simulink model "Final_Model_Building_2_AirflowAdded_BufferMode"  (R2022a)
settings: Solver=FixedStepAuto  StartTime=0.0  StopTime=24*3600  FixedStep=5  RelTol=1e-3
values from neighbouring files (symbols this model uses):
  Aux_Threshold = 52    [Setup_Code_EWASP_VC.m]
  buildingAge = 2005    [Setup_Code_EWASP_VC.m]
  ceilingHeight = 2.4    [Setup_Code_EWASP_VC.m]
  conductiveHconnectMatrix = [ ... (first row only)    [Setup_Code_EWASP_VC.m]
  cRoofGreen = 100000    [Setup_Code_EWASP_VC.m]
  Defrost_After_Time = 30    [Setup_Code_EWASP_VC.m]
  DHWDemandProfile = occFreegainHotwaterElecTestPassiveOcc3(:,3)    [Setup_Code_EWASP_VC.m]
  Elec_Max = Elec_Max*(30/24.2)    [Setup_Code_EWASP_VC.m]
  Elec_Mid = Elec_Mid*(30/24.2)    [Setup_Code_EWASP_VC.m]
  Elec_Min = Elec_Min*(30/24.2)    [Setup_Code_EWASP_VC.m]
  ElecDemandProfile = occFreegainHotwaterElecTestPassiveOcc3(:,4)    [Setup_Code_EWASP_VC.m]
  ElecFixed = [Elec_Max(6,2) Elec_Max(6,4) Elec_Max(6,6) Elec_Max(6,7) ... (first row only)    [Setup_Code_EWASP_VC.m]
  floorOrCeilingArea = floorOrCeilingArea*1.15    [Setup_Code_EWASP_VC.m]
  freegain = occFreegainHotwaterElecTestPassiveOcc3(:,2)-max(occupancy)*25    [Setup_Code_EWASP_VC.m]
  furnitureModelOn = 1    [Setup_Code_EWASP_VC.m]
  Heat_Max = Heat_Max*(30/24.2)    [Setup_Code_EWASP_VC.m]
  Heat_Mid = Heat_Mid*(30/24.2)    [Setup_Code_EWASP_VC.m]
  Heat_Min = Heat_Min*(30/24.2)    [Setup_Code_EWASP_VC.m]
  HeatFixed = [Heat_Max(6,2) Heat_Max(6,4) Heat_Max(6,6) Heat_Max(6,7) ... (first row only)    [Setup_Code_EWASP_VC.m]
  HeatingOnProfile = repmat(HeatingOnProfile,365,1)    [Setup_Code_EWASP_VC.m]
  HEX_ReturnLowerLimit = 52.5    [Setup_Code_EWASP_VC.m]
  HEX_ReturnUpperLimit = 55    [Setup_Code_EWASP_VC.m]
  LeakMultiplier = 1+(2*(rand()-0.5)/10)    [Setup_Code_EWASP_VC.m]
  maxOcc = max(occupancyProfile)    [Setup_Code_EWASP_VC.m]
  NESW_wallArea = max(NESW_Lengths*ceilingHeight-NESW_Windows,0)    [Setup_Code_EWASP_VC.m]
  NESW_Windows = [ ... (first row only)    [Setup_Code_EWASP_VC.m]
  numRooms = roomCount    [Setup_Code_EWASP_VC.m]
  occupancy = occupancyProfile    [Setup_Code_EWASP_VC.m]
  offsetDays = 0    [Setup_Code_EWASP_VC.m]
  overChargeSeries = repmat(overChargeSeries,365,1)    [Setup_Code_EWASP_VC.m]
  pumpChoice = pumpChoices(MinIndex,1)    [Setup_Code_EWASP_VC.m]
  pumpRamp = 180    [Setup_Code_EWASP_VC.m]
  RoofIrradiance = Flat_NS_EW_RoofIrradiance(:,1)    [Setup_Code_EWASP_VC.m]
  roofStartTemp = ones(11,1)*20    [Setup_Code_EWASP_VC.m]
  rooftype = 0    [Setup_Code_EWASP_VC.m]
  RoomDataMatrix = [zeros(1,12);ones(1,12)*wallDensity;zeros(1,12);ones(1,12)*wallU;ones(1,12)*windowU;ones(1,12)*floorU;ones(1,12)*ceilingU;zeros(1,12);windowArea, 0;floorOrCeilingArea;zeros(1,12);floorOrCeilingArea*ceilingHeight]    [Setup_Code_EWASP_VC.m]
  roomVol = roomVol*1.15    [Setup_Code_EWASP_VC.m]
  slabStartTemp = (GroundTempTimeSeries(offsetDays*1440+1,1)+thermostatSetting)/2    [Setup_Code_EWASP_VC.m]
  SlackRequest = zeros(1440,1)    [Setup_Code_EWASP_VC.m]
  SolarThermalExists = 0    [Setup_Code_EWASP_VC.m]
  SourceFixed = HeatFixed-ElecFixed    [Setup_Code_EWASP_VC.m]
  StateSeries = StateSeriesGenerator(22,7,1)    [Setup_Code_EWASP_VC.m]
  Tank_Lower_Temp = 49.5    [Setup_Code_EWASP_VC.m]
  Tank_Upper_Temp = 52    [Setup_Code_EWASP_VC.m]
  Tank_Volume_m3 = 0.15    [Setup_Code_EWASP_VC.m]
  TankHeatHour = randi([1 5])-1    [Setup_Code_EWASP_VC.m]
  upDown = [0;0;0;0;1;1;1;1;1;1;1]    [Setup_Code_EWASP_VC.m]
  wallStartTempExt = thermostatSetting*(0.266+0.00215*outdoorStartTemp+0.018*wallU+0.00113*outdoorStartTemp*wallU+0.0068*wallU^2)    [Setup_Code_EWASP_VC.m]
undefined symbols (not defined in the file or in its folder): a, ceilingU, condUDMatrix, convUDMatrix, deltaPEXPANDED_E, deltaPEXPANDED_E2, deltaPEXPANDED_N, deltaPEXPANDED_N2, deltaPEXPANDED_S, deltaPEXPANDED_S2, deltaPEXPANDED_W, deltaPEXPANDED_W2, DesiredDHWTemp, DesiredFlowTempVsInOutDeltaTemp, DiffuseHorizontal, DiscIntNeverNeededParam, DNI, dwnAndConcrete, ExtractRates, GroundTempTimeSeries, HCM, HCM2, HCM_closed, HCM_closed2, intermediateU, IsTop, massFlowMatrix, mechEfficiency, neighbourMatrix, numericalRoomUse, RadiatorMatrix, room2roomflowmatrix_E, room2roomflowmatrix_E2, room2roomflowmatrix_N, room2roomflowmatrix_N2, room2roomflowmatrix_S, room2roomflowmatrix_S2, room2roomflowmatrix_W, room2roomflowmatrix_W2, StateAirInEXPANDED_E, StateAirInEXPANDED_E2, StateAirInEXPANDED_N, StateAirInEXPANDED_N2, StateAirInEXPANDED_S, StateAirInEXPANDED_S2, StateAirInEXPANDED_W, StateAirInEXPANDED_W2, StateAirOutEXPANDED_E, StateAirOutEXPANDED_E2, StateAirOutEXPANDED_N, StateAirOutEXPANDED_N2, StateAirOutEXPANDED_S, StateAirOutEXPANDED_S2, StateAirOutEXPANDED_W, StateAirOutEXPANDED_W2, tankExists, TemperatureSeries, ThermostatBand, ThermostatSetting, Tin1 ... (+10)
libraries: simulink x6, dspsigops x4, dspmtrx3 x4, powerlib_meascontrol x3, carnot x3, dspstat3 x2
(part 29 of 29)

== matlab function Final_Model_Building_2_AirflowAdded_BufferMode/Subsystem_Room6/Bedroom1/Subsystem3/MATLAB Function ==
  data: uValWall input; deltaTint output; c_InPU input; c_MidPU input; c_OutPU input; T_InWall input; T_MidWall input; T_OutWall input; T_Room input; T_AmbientSeries input; windSpeedSeries input; deltaTmid output; deltaTout output; ceilArea input; roomNumber input; logRoomHeatLoss output; Time input; offsetDays input
function [deltaTint,deltaTmid,deltaTout,logRoomHeatLoss] = fcn(uValWall,c_InPU,c_MidPU,c_OutPU,T_InWall, T_MidWall,T_OutWall,T_Room,T_AmbientSeries,windSpeedSeries,ceilArea,roomNumber,Time,offsetDays)




  deltaTint=zeros(1,1);
   deltaTmid=zeros(1,1);
    deltaTout=zeros(1,1);
    logRoomHeatLoss=zeros(1,1);

    v_Wind=windSpeedSeries(ceil((offsetDays*1440)+Time/60+0.00001),1);
   T_Ambient=T_AmbientSeries(ceil((offsetDays*1440)+Time/60+0.00001),1);
    
k_InMid=uValWall*2;
k_OutMid=uValWall*2;




    
    if ceilArea>0

c_In=c_InPU*ceilArea;
c_Mid=c_MidPU*ceilArea;
c_Out=c_OutPU*ceilArea;

    
aA=[-(k_InMid*ceilArea)/c_In (k_InMid*ceilArea)/c_In 0
 (k_InMid*ceilArea)/c_Mid -((k_InMid+k_OutMid)*ceilArea)/c_Mid (k_OutMid*ceilArea)/c_Mid
 0 (k_OutMid*ceilArea)/c_Out -(k_OutMid*ceilArea)/c_Out];

bA=[1/c_In 0 0
 0 1/c_Mid 0
 0 0 1/c_Out];
    
ab=[T_InWall
    T_MidWall
    T_OutWall];

bb=[(2.5*(T_Room-T_InWall)+5.6*(T_Room-T_InWall))*ceilArea
0    
(2.8+3*v_Wind)*(T_Ambient-T_OutWall)+5.6*(T_Ambient-T_OutWall)*ceilArea];

deltaT=aA*ab+bA*bb;

    deltaTint=deltaT(1,1);
   deltaTmid=deltaT(2,1);
    deltaTout=deltaT(3,1);
    
    logRoomHeatLoss=bb(1,1);
    
    else
        
        deltaTint=0;
   deltaTmid=0;
    deltaTout=0;
        
    logRoomHeatLoss=0;
    
    end

== matlab function Final_Model_Building_2_AirflowAdded_BufferMode/Subsystem_Room6/Bedroom1/Subsystem3/MATLAB Function1 ==
  data: Time input; offsetDays input; SurfaceAlbedo input; Tot_Irradiance output; RoofArea input; c_OutRoof input; deltaTexternal output; RoofIrradiance input
function [Tot_Irradiance, deltaTexternal] = SolarSeriesToExtWallGains(Time,offsetDays,SurfaceAlbedo,RoofArea,c_OutRoof,RoofIrradiance)

PU_AreaIrr=RoofIrradiance(ceil((offsetDays*1440)+Time/60+0.00001),1)/2;%extracts correct Diff for the timestep, factor of 1/2 corrects for 90 degree walls (so only half Diff irradiance can be utilised)


Tot_Irradiance=(RoofArea*PU_AreaIrr)*(1-SurfaceAlbedo);
deltaTexternal=Tot_Irradiance./(c_OutRoof*RoofArea);

    
end

== matlab function Final_Model_Building_2_AirflowAdded_BufferMode/Subsystem_Room2/Kitchen/Subsystem3/MATLAB Function ==
  data: uValWall input; deltaTint output; c_InPU input; c_MidPU input; c_OutPU input; T_InWall input; T_MidWall input; T_OutWall input; T_Room input; T_AmbientSeries input; windSpeedSeries input; deltaTmid output; deltaTout output; ceilArea input; roomNumber input; logRoomHeatLoss output; Time input; offsetDays input
function [deltaTint,deltaTmid,deltaTout,logRoomHeatLoss] = fcn(uValWall,c_InPU,c_MidPU,c_OutPU,T_InWall, T_MidWall,T_OutWall,T_Room,T_AmbientSeries,windSpeedSeries,ceilArea,roomNumber,Time,offsetDays)




  deltaTint=zeros(1,1);
   deltaTmid=zeros(1,1);
    deltaTout=zeros(1,1);
    logRoomHeatLoss=zeros(1,1);

    v_Wind=windSpeedSeries(ceil((offsetDays*1440)+Time/60+0.00001),1);
   T_Ambient=T_AmbientSeries(ceil((offsetDays*1440)+Time/60+0.00001),1);
    
k_InMid=uValWall*2;
k_OutMid=uValWall*2;




    
    if ceilArea>0

c_In=c_InPU*ceilArea;
c_Mid=c_MidPU*ceilArea;
c_Out=c_OutPU*ceilArea;

    
aA=[-(k_InMid*ceilArea)/c_In (k_InMid*ceilArea)/c_In 0
 (k_InMid*ceilArea)/c_Mid -((k_InMid+k_OutMid)*ceilArea)/c_Mid (k_OutMid*ceilArea)/c_Mid
 0 (k_OutMid*ceilArea)/c_Out -(k_OutMid*ceilArea)/c_Out];

bA=[1/c_In 0 0
 0 1/c_Mid 0
 0 0 1/c_Out];
    
ab=[T_InWall
    T_MidWall
    T_OutWall];

bb=[(2.5*(T_Room-T_InWall)+5.6*(T_Room-T_InWall))*ceilArea
0    
(2.8+3*v_Wind)*(T_Ambient-T_OutWall)+5.6*(T_Ambient-T_OutWall)*ceilArea];

deltaT=aA*ab+bA*bb;

    deltaTint=deltaT(1,1);
   deltaTmid=deltaT(2,1);
    deltaTout=deltaT(3,1);
    
    logRoomHeatLoss=bb(1,1);
    
    else
        
        deltaTint=0;
   deltaTmid=0;
    deltaTout=0;
        
    logRoomHeatLoss=0;
    
    end
